simulink model "motorModel"  (R2015a)
settings: Solver=ode45  StartTime=0.0  StopTime=20  RelTol=1e-3
values from neighbouring files (symbols this model uses):
  b = 0.1    [motorModel.mat]
  J = 0.01    [motorModel.mat]
  K = 0.01    [motorModel.mat]
  L = 0.5    [motorModel.mat]
  R = 1    [motorModel.mat]
undefined symbols (not defined in the file or in its folder): Kd, Ki, Kp
settings Model: Creator=tabdallah1518  LastModifiedBy=tabdallah1518

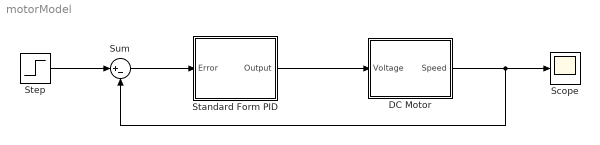
== system motorModel ==
  DC Motor : Subsystem
  Scope : Scope
  Standard Form PID : Subsystem
  Step : Step  Time=0  SampleTime=0
  Sum : Sum  Inputs=|+-
  wires:
  DC Motor/1(Speed) -> Sum/2, Scope/1
  Standard Form PID/1(Output) -> DC Motor/1(Voltage)
  Step/1 -> Sum/1
  Sum/1 -> Standard Form PID/1(Error)

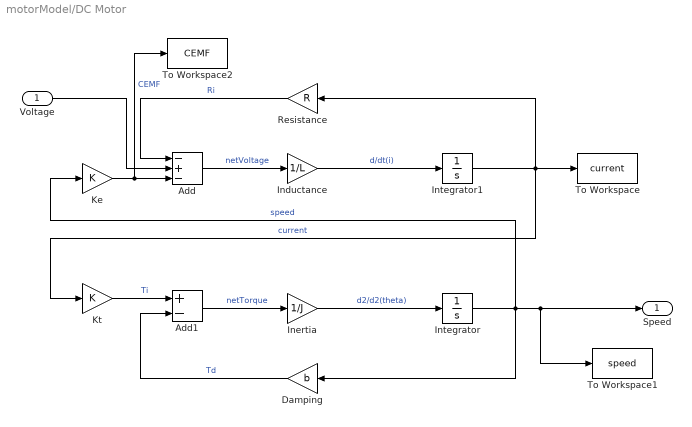
== system motorModel/DC Motor ==
  Voltage : Inport
  Add : Sum  Inputs=-+-
  Add1 : Sum  Inputs=+-
  Damping : Gain  Gain=b
  Inductance : Gain  Gain=1/L
  Inertia : Gain  Gain=1/J
  Integrator : Integrator
  Integrator1 : Integrator
  Ke : Gain  Gain=K
  Kt : Gain  Gain=K
  Resistance : Gain  Gain=R
  To Workspace : ToWorkspace  VariableName=current  SaveFormat=Timeseries  SampleTime=-1
  To Workspace1 : ToWorkspace  VariableName=speed  SaveFormat=Timeseries  SampleTime=-1
  To Workspace2 : ToWorkspace  VariableName=CEMF  SaveFormat=Timeseries  SampleTime=-1
  Speed : Outport
  wires:
  Add1/1 -> Inertia/1  "netTorque"
  Inertia/1 -> Integrator/1  "d2/d2(theta)"
  Integrator1/1 -> To Workspace/1, Resistance/1, Kt/1  "current"
  Integrator/1 -> To Workspace1/1, Speed/1, Ke/1, Damping/1  "speed"
  Inductance/1 -> Integrator1/1  "d/dt(i)"
  Add/1 -> Inductance/1  "netVoltage"
  Damping/1 -> Add1/2  "Td"
  Resistance/1 -> Add/1  "Ri"
  Kt/1 -> Add1/1  "Ti"
  Ke/1 -> To Workspace2/1, Add/3  "CEMF"
  Voltage/1 -> Add/2

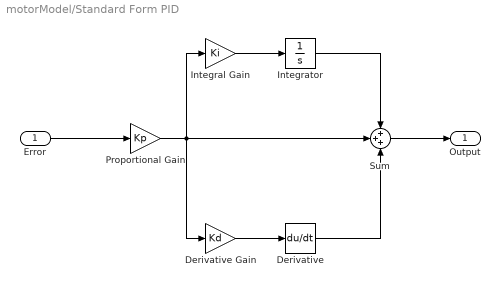
== system motorModel/Standard Form PID ==
  Error : Inport
  Derivative : Derivative
  Derivative Gain : Gain  Gain=Kd
  Integral Gain : Gain  Gain=Ki
  Integrator : Integrator
  Proportional Gain : Gain  Gain=Kp
  Sum : Sum  Inputs=+++
  Output : Outport
  wires:
  Error/1 -> Proportional Gain/1
  Derivative/1 -> Sum/3
  Integrator/1 -> Sum/1
  Proportional Gain/1 -> Integral Gain/1, Derivative Gain/1, Sum/2
  Sum/1 -> Output/1
  Derivative Gain/1 -> Derivative/1
  Integral Gain/1 -> Integrator/1
